simulink model "interp_1"  (Simulink 4.00)
settings: Solver=ode45  StartTime=0.0  StopTime=10.0  RelTol=1e-3
libraries: simulink3 x5
settings Model: LastModifiedBy=Administrator  BlockReductionOpt=off

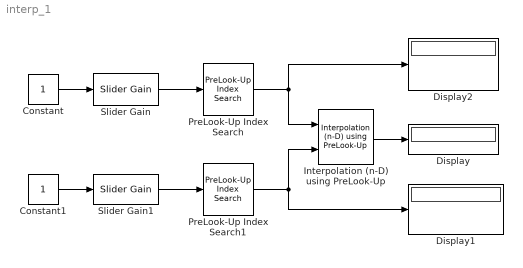
== system interp_1 ==
  Constant : Constant  Value=1
  Constant1 : Constant  Value=1
  Display : Display
      settings: Format=short
  Display1 : Display
      settings: Format=short
  Display2 : Display
      settings: Format=short
  Interpolation (n-D) using PreLook-Up : simulink3/Functions & Tables/Interpolation (n-D) using PreLook-Up  numDimsPopupSelect=2  explicitNumDims=2  table=sqrt([1:10]'*[1:10])  interpMethod=Linear  extrapMethod=Linear  rangeErrorMode=None
  PreLook-Up Index Search : simulink3/Functions & Tables/PreLook-Up Index Search  bpData=[5:14]  searchMode=Binary Search  cacheBpFlag=off  outputFlag=off  extrapMode=Linear Extrapolation  rangeErrorMode=None
  PreLook-Up Index Search1 : simulink3/Functions & Tables/PreLook-Up Index Search  bpData=[20:10:110]  searchMode=Binary Search  cacheBpFlag=off  outputFlag=off  extrapMode=Linear Extrapolation  rangeErrorMode=None
  Slider Gain : simulink3/Math/Slider Gain  low=5  gain=8.48  high=14
  Slider Gain1 : simulink3/Math/Slider Gain  low=20  gain=76.34  high=110
  wires:
  PreLook-Up Index Search/1 -> Interpolation (n-D) using PreLook-Up/1, Display2/1
  PreLook-Up Index Search1/1 -> Interpolation (n-D) using PreLook-Up/2, Display1/1
  Interpolation (n-D) using PreLook-Up/1 -> Display/1
  Constant/1 -> Slider Gain/1
  Slider Gain/1 -> PreLook-Up Index Search/1
  Constant1/1 -> Slider Gain1/1
  Slider Gain1/1 -> PreLook-Up Index Search1/1
